simulink model "lstm_test_data"  (R2018a)
settings: Solver=ode45  StartTime=0.0  StopTime=30000  RelTol=1e-3
settings Model: Creator=User  LastModifiedBy=nfm
settings DataIOCC: ReturnWorkspaceOutputs=on
settings SFSimCC: SimUseLocalCustomCode=on
settings RTWCC: RTWUseLocalCustomCode=on

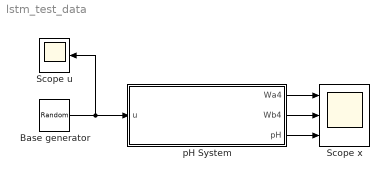
== system lstm_test_data ==
  " pH System " : Subsystem
  Base generator : UniformRandomNumber  Minimum=0  Maximum=50  Seed=7  SampleTime=50
  Scope u : Scope
  Scope x : Scope  NumInputPorts=3
  wires:
  " pH System "/1(Wa4) -> Scope x/1
  " pH System "/2(Wb4) -> Scope x/2
  " pH System "/3(pH) -> Scope x/3
  Base generator/1 -> Scope u/1, " pH System "/1(u)

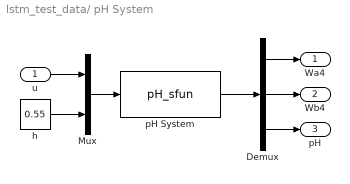
== system lstm_test_data/ pH System  ==
  u : Inport
  " h " : Constant  Value=0.55
  Demux : Demux  Outputs=3
  Mux : Mux  Inputs=2
  pH System : S-Function  FunctionName=pH_sfun  SFunctionDeploymentMode=off  EnableBusSupport=off
  Wa4 : Outport
  Wb4 : Outport  Port=2
  pH : Outport  Port=3
  wires:
  Mux/1 -> pH System/1
  pH System/1 -> Demux/1
  u/1 -> Mux/1
  Demux/2 -> Wb4/1
  Demux/1 -> Wa4/1
  Demux/3 -> pH/1
  " h "/1 -> Mux/2
